simulink model "alsomitra_RL3"  (R2024a)
settings: Solver=ode3  StartTime=0.0  StopTime=14  FixedStep=0.1  RelTol=1e-3
libraries: rllib x1
settings Model: Creator=Colin Kessler  LastModifiedBy=Colin Kessler
settings SolverCC: AllowMultiTaskInputOutput=on  ConcurrentTasks=on  AutoInsertRateTranBlk=on
settings DataIOCC: SaveFormat=Array  SaveState=on  StateSaveName=dx_dt

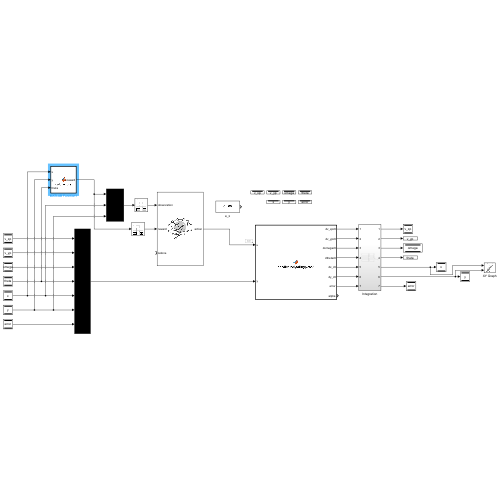
[thumbnail: Simulink's stored preview of the top-level diagram]
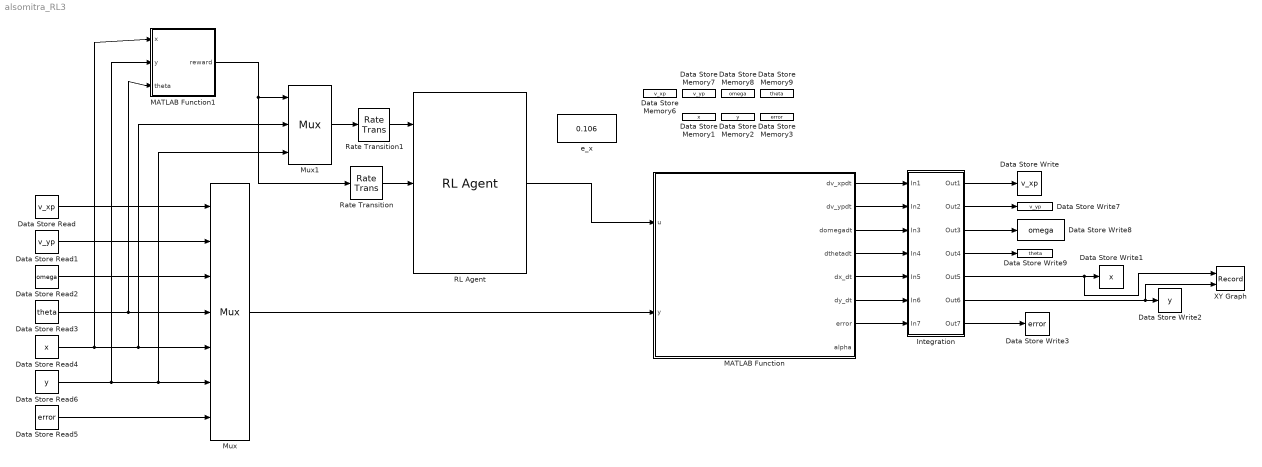
== system alsomitra_RL3 ==
  Data Store Memory1 : DataStoreMemory  DataStoreName=x  WriteAfterWriteMsg=warning  ShowAdditionalParam=off
  Data Store Memory2 : DataStoreMemory  DataStoreName=y  WriteAfterWriteMsg=warning  ShowAdditionalParam=off
  Data Store Memory3 : DataStoreMemory  DataStoreName=error  WriteAfterWriteMsg=warning  ShowAdditionalParam=off
  Data Store Memory6 : DataStoreMemory  DataStoreName=v_xp  WriteAfterWriteMsg=warning  InitialValue=1  ShowAdditionalParam=off
  Data Store Memory7 : DataStoreMemory  DataStoreName=v_yp  WriteAfterWriteMsg=warning  ShowAdditionalParam=off
  Data Store Memory8 : DataStoreMemory  DataStoreName=omega  WriteAfterWriteMsg=warning  ShowAdditionalParam=off
  Data Store Memory9 : DataStoreMemory  DataStoreName=theta  WriteAfterWriteMsg=warning  InitialValue=0.1  ShowAdditionalParam=off
  Data Store Read : DataStoreRead  DataStoreName=v_xp  IndexOptions=Index vector (dialog)  Indices=1  OutputSizes=1
  Data Store Read1 : DataStoreRead  DataStoreName=v_yp  IndexOptions=Index vector (dialog)  Indices=1  OutputSizes=1
  Data Store Read2 : DataStoreRead  DataStoreName=omega  IndexOptions=Index vector (dialog)  Indices=1  OutputSizes=1
  Data Store Read3 : DataStoreRead  DataStoreName=theta  IndexOptions=Index vector (dialog)  Indices=1  OutputSizes=1
  Data Store Read4 : DataStoreRead  DataStoreName=x  IndexOptions=Index vector (dialog)  Indices=1  OutputSizes=1
  Data Store Read5 : DataStoreRead  DataStoreName=error  IndexOptions=Index vector (dialog)  Indices=1  OutputSizes=1
  Data Store Read6 : DataStoreRead  DataStoreName=y  IndexOptions=Index vector (dialog)  Indices=1  OutputSizes=1
  Data Store Write : DataStoreWrite  DataStoreName=v_xp  IndexOptions=Index vector (dialog)  Indices=1  OutputSizes=1
  Data Store Write1 : DataStoreWrite  DataStoreName=x  IndexOptions=Index vector (dialog)  Indices=1  OutputSizes=1
  Data Store Write2 : DataStoreWrite  DataStoreName=y  IndexOptions=Index vector (dialog)  Indices=1  OutputSizes=1
  Data Store Write3 : DataStoreWrite  DataStoreName=error  IndexOptions=Index vector (dialog)  Indices=1  OutputSizes=1
  Data Store Write7 : DataStoreWrite  DataStoreName=v_yp  IndexOptions=Index vector (dialog)  Indices=1  OutputSizes=1
  Data Store Write8 : DataStoreWrite  DataStoreName=omega  IndexOptions=Index vector (dialog)  Indices=1  OutputSizes=1
  Data Store Write9 : DataStoreWrite  DataStoreName=theta  IndexOptions=Index vector (dialog)  Indices=1  OutputSizes=1
  Integration : Subsystem
  MATLAB Function : MATLAB Function  TreatAsAtomicUnit=on
  MATLAB Function1 : MATLAB Function  TreatAsAtomicUnit=on
  Mux : Mux  Inputs=7
  Mux1 : Mux  Inputs=3
  RL Agent : rllib/RL Agent  Agent=agentObj  ExternalActionAsInput=off  ProvideLastAction=off  ProvideCumRwd=off  TreatAsDirectFeedthrough=on  UseStrictObservationDataTypes=off
  Rate Transition : RateTransition
  Rate Transition1 : RateTransition
  XY Graph : Record  FileSettingsInternal="{\"entries\":[{\"content\":{\"excelSettings\":{\"content\":{},\"type\":\"Streamout.ExcelSettings\"}},\"type\":\"Streamout.FileSettingStorage\",\"uuid\":\"\"}],\"packageUris\":[\"http:\\/\\/schema.mathworks.com\\/mf0\\/streamout_blocks\\/R2020a\"],\"version\":\"1.0\"}"  Layout=[1 1]  SignalsInternal="{\"entries\":[{\"content\":{\"signals\":[{\"content\":{\"blockPath\":[],\"dimensions\":[1],\"domain\":\"\",\"lineColor\":\"#a2142f\",\"plots\":[ 1 ],\"port\":1,\"sid\":[\"\"],\"signalID\":1,\"signalName\":\"Integration:5\"},\"type\":\"RecordBlkView.Signal\",\"uuid\":\"\"},{\"content\":{\"blockPath\":[],\"dimensions\":[1],\"domain\":\"\",\"lineColor\":\"#139fff\",\"plots\":[ 1 ],\"port\":2,\"sid\":[\"\"],\"signalID\":2,\"signalName\":\"Integration:6\"},\"type\":\"RecordBlkView.Signal\",\"uuid\":\"\"}]},\"type\":\"RecordBlkView.InputSignals\",\"uuid\":\"\"}],\"packageUris\":[\"http:\\/\\/schema.mathworks.com\\/mf0\\/streamout_blocks\\/R2020a\"],\"version\":\"1.0\"}"  VisualizationBindings="{\"xyplotplugin\":{\"info\":[{\"series\":[{\"bindingParametersList\":[{\"parameter\":\"X-Axis\",\"signalID\":1,\"signalName\":\"Integration:5\"},{\"parameter\":\"Y-Axis\",\"signalID\":2,\"signalName\":\"Integration:6\"}],\"seriesID\":0}],\"subplotID\":1}]}}"  CompatibilityTag=XY
  e_x : Constant  Value=0.106
  wires:
  Data Store Read5/1 -> Mux/7
  Data Store Read6/1 -> MATLAB Function1/2(y), Mux1/3, Mux/6
  Data Store Read4/1 -> MATLAB Function1/1(x), Mux1/2, Mux/5
  Data Store Read3/1 -> MATLAB Function1/3(theta), Mux/4
  Data Store Read2/1 -> Mux/3
  Data Store Read1/1 -> Mux/2
  Data Store Read/1 -> Mux/1
  Mux/1 -> MATLAB Function/2(y)
  Integration/6(Out6) -> XY Graph/2, Data Store Write2/1
  Integration/5(Out5) -> XY Graph/1, Data Store Write1/1
  MATLAB Function/1(dv_xpdt) -> Integration/1(In1)
  MATLAB Function/2(dv_ypdt) -> Integration/2(In2)
  MATLAB Function/3(domegadt) -> Integration/3(In3)
  MATLAB Function/4(dthetadt) -> Integration/4(In4)
  MATLAB Function/5(dx_dt) -> Integration/5(In5)
  MATLAB Function/6(dy_dt) -> Integration/6(In6)
  MATLAB Function/7(error) -> Integration/7(In7)
  Integration/1(Out1) -> Data Store Write/1
  Integration/2(Out2) -> Data Store Write7/1
  Integration/3(Out3) -> Data Store Write8/1
  Integration/4(Out4) -> Data Store Write9/1
  Integration/7(Out7) -> Data Store Write3/1
  MATLAB Function1/1(reward) -> Mux1/1, Rate Transition/1
  RL Agent/1 -> MATLAB Function/1(u)
  Mux1/1 -> Rate Transition1/1
  Rate Transition/1 -> RL Agent/2
  Rate Transition1/1 -> RL Agent/1

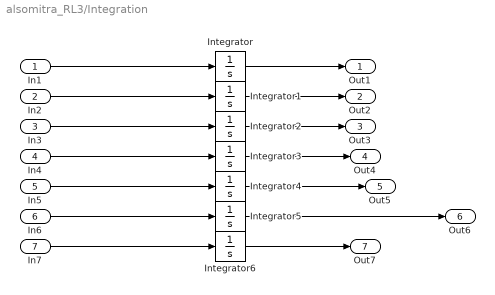
== system alsomitra_RL3/Integration ==
  In1 : Inport
  In2 : Inport  Port=2
  In3 : Inport  Port=3
  In4 : Inport  Port=4
  In5 : Inport  Port=5
  In6 : Inport  Port=6
  In7 : Inport  Port=7
  Integrator{,1..6} (7 alike) : Integrator
  Out1 : Outport
  Out2 : Outport  Port=2
  Out3 : Outport  Port=3
  Out4 : Outport  Port=4
  Out5 : Outport  Port=5
  Out6 : Outport  Port=6
  Out7 : Outport  Port=7
  wires:
  Integrator1/1 -> Out2/1
  In2/1 -> Integrator1/1
  In4/1 -> Integrator3/1
  In6/1 -> Integrator5/1
  In3/1 -> Integrator2/1
  In5/1 -> Integrator4/1
  In7/1 -> Integrator6/1
  Integrator/1 -> Out1/1
  Integrator5/1 -> Out6/1
  Integrator2/1 -> Out3/1
  Integrator4/1 -> Out5/1
  Integrator3/1 -> Out4/1
  In1/1 -> Integrator/1
  Integrator6/1 -> Out7/1

== matlab function alsomitra_RL3/MATLAB Function1 ==
  data: x input; reward output; y input; theta input
function reward  = calc_errors(x,y,theta)

    % Target trajectory
    x_c1 = -0.5:0.1:4.5;
    y_c1 = -x_c1;
    y_c2 = -4.6:-0.1:-6.5;
    x_c2 = sqrt(2-((y_c2+5.5).^2))+3.5;
    x_c3 = 4.4:-0.1:3.5;
    y_c3 = x_c3 - 11;
    y_c4 = -7.6:-0.1:-9.5;
    x_c4 = -sqrt(2-((y_c4+8.5).^2))+4.5;
    x_c5 = 3.6:0.1:10;
    y_c5 = -x_c5 - 6;
    x_c1 = [x_c1,x_c2,x_c3,x_c4,x_c5]/5 * 1000/70;
    y_c1 = [y_c1,y_c2,y_c3,y_c4,y_c5]/5 * 1000/70;

    distances1 = ((x_c1-x).^2);
    distances2 = ((y_c1-y).^2);
    [val,idx] = min(distances1+distances2);

    theta2 = atan2((y_c1(idx+1)-y_c1(idx-1)),(x_c1(idx+1)-x_c1(idx-1)));
    intercept2 = y_c1(idx) - (tan(theta2) * x_c1(idx));
    intercept = y - (tan(theta-pi/2)*x);

    xt = (intercept2-intercept)/ (tan(theta-pi/2)- tan(theta2));
    yt = tan(theta-pi/2)*xt + intercept;

    thetat = theta2;

    e1x = x - xt;
    e1y = y - yt;
    e1 = sqrt((e1x^2)+(e1y^2)) * - (abs(e1y)/e1y);

    if abs(e1) < 0.1
        e1 = 0.1;
    end

    e2 = theta - thetat;

    if abs(e2) < 0.1
        e2 = 0.1;
    end

    reward = 1/(abs(e1)) + 1/(abs(e2));
end

== matlab function alsomitra_RL3/MATLAB Function ==
  data: u input; y input; dv_xpdt output; dv_ypdt output; domegadt output; dthetadt output; dx_dt output; dy_dt output; error output; alpha output
function [dv_xpdt, dv_ypdt, domegadt, dthetadt, dx_dt, dy_dt, error, alpha] = nondimfreelyfallingplate3(u,y)
    
    % global p %p_aero 
    p_aero = [5.18218452125279	0.807506506794260	0.105977518471870	4.93681162104530	1.49958010664229	0.238565281050545	2.85289007725274	0.368933365279324	1.73001889433847];


    % Extract v_xp, v_yp, omega, theta x_ and y_ from input vector y
    v_xp = y(1);
    v_yp = y(2);
    omega = y(3);
    theta = y(4);
    x_ = y(5);
    y_ = y(6);
    error_ = y(7);

    p = [0.070000000000000;3.175000000000000e-04;1.225000000000000;0.033750000000000;5.000000000000000e-04;0.174500000000000];
    l = p(1);
    m = p(2);
    rho_f = p(3);
    a = p(4);
    b = p(5);
    s = p(6);

    rho_s = m/(pi*a*b);
    %h = m/(rho_s*l);

    C_L1 = p_aero(1);
    C_L2 = p_aero(2);
    C_D0 = p_aero(3);
    C_D1 = p_aero(4);
    C_D_pi_2 = p_aero(5);
    C_0_CP = p_aero(6);
    C_1_CP = p_aero(7);
    C_2_CP = p_aero(8);
    C_R = p_aero(9);
    e_x= u(1);

    % l_CM = l_CE*(rho_s - rho_f)/rho_s; 
    l_CM = e_x * l;
    % % U = 2*sqrt(((rho_s/rho_f)-1)*(h*g/pi));
    
    m_prime = 4 * m / (pi * rho_f * l * l * s);
    % m_prime = 4*rho_s*l*0.001/(pi*rho_f*l);
    % m_prime = 33.0329;
    % m_prime = 5.7642;
    % m_prime = 2.9103;
    % m_prime = 0.5853;

    % Cathal's plot on Slack 14/06/23
    % beta = h/l;
    % gamma = rho_f/(rho_s-rho_f);
    % alpha depends on time t

    % From Cathal 27/03/24
    % beta = 0.001;
    % beta = b/l;
    %gamma = 0.0029;
    gamma = rho_f/(rho_s-rho_f);

    alpha = atan2((v_yp),v_xp); 
    % alpha = atan2((v_yp - omega*l_CM),v_xp); 
    % alpha = atan((v_yp)/v_xp); 
    
    % critical angle of attack at stall
    alpha0 = deg2rad(14);
    % delta is the smoothness of the transition from laminar to turbulent
    delta = deg2rad(6);

    % f activation function, it specifies laminar and stall regimes
    Falpha1 = ((1 - tanh((pi - abs(alpha) - alpha0)/delta))/2);
    Falpha2 = ((1 - tanh((abs(alpha) - alpha0)/delta))/2);
    Falpha3 = ((1 - tanh((alpha - alpha0)/delta))/2);
    Falpha4 = ((1 - tanh((pi - alpha - alpha0)/delta))/2);
    % Falpha = Falpha1.*(alpha>=-pi & alpha<=-pi/2) + Falpha2.*(alpha>=-pi/2 & alpha<=0) + Falpha3.*(alpha>=0 & alpha<=pi/2) + Falpha4.*(alpha>=pi/2 & alpha<=pi);

    % C_Lalpha = Falpha*C_L1.*sin(alpha) + (1-Falpha)*C_L2.*sin(2*alpha);
    C_Lalpha1 = Falpha1*C_L1.*sin(pi - abs(alpha)) + (1-Falpha1)*C_L2.*sin(2*(pi - abs(alpha)));
    C_Lalpha2 = Falpha2*C_L1.*sin(abs(alpha)) + (1-Falpha2)*C_L2.*sin(2*abs(alpha));
    C_Lalpha3 = Falpha3*C_L1.*sin(alpha) + (1-Falpha3)*C_L2.*sin(2*alpha);
    C_Lalpha4 = Falpha4*C_L1.*sin(pi - alpha) + (1-Falpha4)*C_L2.*sin(2*(pi - alpha));
    C_Lalpha = C_Lalpha1.*(alpha>=-pi & alpha<=-pi/2) - C_Lalpha2.*(alpha>-pi/2 & alpha<=0) + C_Lalpha3.*(alpha>0 & alpha<=pi/2) - C_Lalpha4.*(alpha>pi/2 & alpha<=pi);

    % C_Dalpha = Falpha.*(C_D0 + C_D1.*sin((alpha).^2)) + (1 - Falpha).*C_D_pi_2.*(sin(alpha).^2);
    C_Dalpha1 = Falpha1.*(C_D0 + C_D1.*sin((pi - abs(alpha)).^2)) + (1 - Falpha1).*C_D_pi_2.*(sin(pi - abs(alpha)).^2);
    C_Dalpha2 = Falpha2.*(C_D0 + C_D1.*sin((abs(alpha)).^2)) + (1 - Falpha2).*C_D_pi_2.*(sin(abs(alpha)).^2);
    C_Dalpha3 = Falpha3.*(C_D0 + C_D1.*sin((alpha).^2)) + (1 - Falpha3).*C_D_pi_2.*(sin(alpha).^2);
    C_Dalpha4 = Falpha4.*(C_D0 + C_D1.*sin((pi - alpha).^2)) + (1 - Falpha4).*C_D_pi_2.*(sin(pi - alpha).^2);
    C_Dalpha = C_Dalpha1.*(alpha>=-pi & alpha<-pi/2) + C_Dalpha2.*(alpha>=-pi/2 & alpha<0) + C_Dalpha3.*(alpha>=0 & alpha<pi/2) + C_Dalpha4.*(alpha>=pi/2 & alpha<=pi);

    % l_CP_alpha_l = Falpha.*(C_0_CP - C_1_CP.*alpha.^2) + (1-Falpha).*C_2_CP.*(1-alpha/(pi/2));
    l_CP_alpha_l1 = Falpha1.*(C_0_CP - C_1_CP.*(pi - abs(alpha)).^2) + (1-Falpha1).*C_2_CP.*(1-(pi - abs(alpha))/(pi/2));
    l_CP_alpha_l2 = Falpha2.*(C_0_CP - C_1_CP.*abs(alpha).^2) + (1-Falpha2).*C_2_CP.*(1-abs(alpha)/(pi/2));
    l_CP_alpha_l3 = Falpha3.*(C_0_CP - C_1_CP.*alpha.^2) + (1-Falpha3).*C_2_CP.*(1-alpha/(pi/2));
    l_CP_alpha_l4 = Falpha4.*(C_0_CP - C_1_CP.*(pi - alpha).^2) + (1-Falpha4).*C_2_CP.*(1-(pi - alpha)/(pi/2));
   
    epsilon_alpha = -l_CP_alpha_l1.*(alpha>=-pi & alpha<=-pi/2) + l_CP_alpha_l2.*(alpha>=-pi/2 & alpha<=0) + l_CP_alpha_l3.*(alpha>=0 & alpha<=pi/2) - l_CP_alpha_l4.*(alpha>=pi/2 & alpha<=pi);

    %% CHECK the following equations are all checked with syms Matlab, in the
    % online course https://matlabacademy.mathworks.com/R2020a/portal.html?course=symbolic#chapter=8&lesson=1&section=1
    % you can type the symbolic equation and get a graphical representation
    % as in Latex.
    
    L_Txy = (2/pi)*C_Lalpha.*sqrt(v_xp^2 + (v_yp - omega*e_x)^2);
    L_Tx = L_Txy.*(v_yp - omega*e_x);
    L_Ty = L_Txy.*(-v_xp);
    % L_T = L_Tx + L_Ty;
  
    L_Rxy = (-2/pi)*C_R*omega;
    L_Rx = L_Rxy*(v_yp - omega*e_x);
    L_Ry = L_Rxy*(-v_xp);
    % L_R = L_Rx + L_Ry;

    % L = L_T + L_R;

    D_xy = (-2/pi)*C_Dalpha*sqrt(v_xp^2 + (v_yp - omega*e_x)^2);
    D_x = D_xy*v_xp;
    D_y = D_xy*(v_yp - omega*e_x);
    % D = D_x + D_y;
    
    % plus sign applies for 2*l_CM/l < 1, when the CoM lies within the plate
    e_xplus = (2*e_x + 1).^4 + (2*e_x - 1).^4;
    e_xminus = (2*e_x + 1).^4 - (2*e_x - 1).^4;

    % if 2*e_x <= 1 

        plus_minus = e_xplus + e_xminus;
    % else
    % 
    %     plus_minus = e_xplus - e_xminus;
    % end
    % 

    Inertia = (m * (a^2 + b^2)/(rho_f * l^4))+1/32+e_x^2;
    
    domegadt = ((-C_D_pi_2/(32*pi))*omega*abs(omega)*plus_minus + ((L_Ty + D_y)*(epsilon_alpha - e_x)) - gamma*e_x*cos(theta))/Inertia;
    
    dv_xpdt = (1/m_prime)*((m_prime + 1)*omega*v_yp - e_x*omega^2 + (L_Tx + L_Rx) + D_x - sin(theta)); 

    dv_ypdt = (1/(m_prime+1))*(-m_prime*omega*v_xp +domegadt*e_x + (L_Ty + L_Ry) + D_y - cos(theta));
    
    dthetadt = omega; 

    dx_dt = v_xp.*cos(theta) - v_yp.*sin(theta);
    
    dy_dt = v_xp.*sin(theta) + v_yp.*cos(theta);

    error = ((y_+dy_dt) * 0.07) - (-1*0.07*(x_+dx_dt)) - error_;

    % dydt = [dv_xpdt; dv_ypdt; domegadt; dthetadt; dx_dt; dy_dt; error; alpha];
end
